simulink model "grasp_object"  (R2019a)
settings: Solver=FixedStepDiscrete  StartTime=0.0  StopTime=inf  FixedStep=0.001  RelTol=1e-3  EnableMultiTasking=on
PreLoadFcn:
  | demos_common_configs();
libraries: franka_simulink_library_misc x5, franka_simulink_library x3, simulink x1
settings Model: SimulationMode=external  ExtModeTrigDuration=10000  Creator=vasi_ko  LastModifiedBy=kvasios
settings DataIOCC: LimitDataPoints=on  SaveFormat=Array  ReturnWorkspaceOutputs=off
settings OptimizationCC: DefaultParameterBehavior=Inlined  EnhancedBackFolding=on  PassReuseOutputArgsAs=Individual arguments  ZeroExternalMemoryAtStartup=off  ZeroInternalMemoryAtStartup=off  OptimizeBlockOrder=speed  DifferentSizesBufferReuse=on  OptimizationCustomize=off
settings DebuggingCC: SolverPrmCheckMsg=warning  ParameterTunabilityLossMsg=error  SFUnexpectedBacktrackingDiag=warning  SFNoUnconditionalDefaultTransitionDiag=warning  SFExecutionAtInitializationDiag=none  ArithmeticOperatorsInVariantConditions=warning
settings HardwareCC: ProdBitPerLong=64  ProdHWDeviceType=Intel->x86-64 (Linux 64)
settings ModelReferenceCC: PropagateSignalLabelsOutOfModel=off
settings SFSimCC: SimUseLocalCustomCode=off  MATLABDynamicMemAlloc=off
settings RTWCC: SystemTargetFile=franka_emika_panda.tlc  GenCodeOnly=on  TemplateMakefile=ert_default_tmf  RTWVerbose=off  RTWUseLocalCustomCode=off  Toolchain=Franka Simulink | gmake (64-bit linux)  BuildConfiguration=Faster Runs  IncludeHyperlinkInReport=on  TargetLang=C++
settings CodeAppCC: ForceParamTrailComments=on  IgnoreCustomStorageClasses=off  OperatorAnnotations=on  SimulinkDataObjDesc=on  SFDataObjDesc=on  InsertBlockDesc=on
settings STFCustomTargetCC: TargetLangStandard=C99 (ISO)  MultiwordLength=256  GenerateSampleERTMain=on  ModelReferenceCompliant=off  CombineOutputUpdateFcns=on  ERTCustomFileBanners=on  SupportNonInlinedSFcns=off  RemoveResetFunc=on  MATLABClassNameForMDSCustomization=Simulink.SoftwareTarget.ERTCustomization  CPPClassGenCompliant=on  GRTInterface=off  UseToolchainInfoCompliant=on  SystemTargetFile=franka_emika_panda.tlc
settings ERTTargetCC: TargetLangStandard=C99 (ISO)  GenerateSampleERTMain=on  ModelReferenceCompliant=off  ParMdlRefBuildCompliant=off  CompOptLevelCompliant=off  ConcurrentExecutionCompliant=off  SupportContinuousTime=on  ModelStepFunctionPrototypeControlCompliant=off  InlinedParameterPlacement=NonHierarchical  ERTCustomFileTemplate=franka_emika_panda_file_process.tlc
settings ConfigComp: CovMetricSettings=dw  CovSaveCumulativeToWorkspaceVar=on  CovSaveSingleToWorkspaceVar=on  CovExternalEMLEnable=off  CovSFcnEnable=off

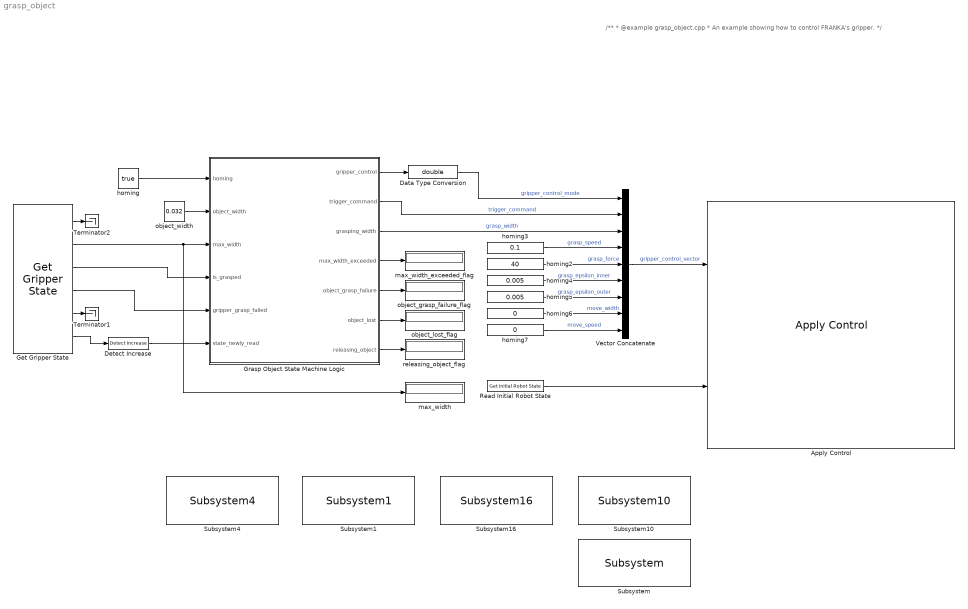
== system grasp_object ==
  note: /**
      |  * @example grasp_object.cpp
      |  * An example showing how to control FRANKA's gripper.
      |  */
  Apply Control : franka_simulink_library/Apply Control  robot_ip=robot_ip  gripper_attached=on  control_mode=Joint Positions - Internal Controller Mode  controller_choice=Joint Impedance Controller  elbow_control=on  collision_thresholds=100*ones(1,52)  joint_impedance=joint_impedance  cartesian_impedance=cartesian_impedance  load_inertia=load_inertia  EE_T_K=EE_T_K  init_joint_configuration_req=off  init_joint_configuration=q_init
      settings: SourceProductName=Franka Emika
  Data Type Conversion : DataTypeConversion  OutDataTypeStr=double
  Detect Increase : simulink/Logic and Bit Operations/Detect Increase  vinit=0.0  OutDataTypeStr=boolean
  Get Gripper State : franka_simulink_library/Get Gripper State  robot_ip=robot_ip
      settings: SourceProductName=Franka Emika
  Grasp Object State Machine Logic : Stateflow chart  TreatAsAtomicUnit=on
  Read Initial Robot State : franka_simulink_library/Get Initial Robot State  robot_ip=robot_ip  signals_requested='q_d'
      settings: SourceProductName=Franka Emika
  Subsystem : franka_simulink_library_misc/Subsystem  SystemSampleTime=-1  Latency=0  AutoFrameSizeCalculation=off
  Subsystem1 : franka_simulink_library_misc/Subsystem1  SystemSampleTime=-1  Latency=0  AutoFrameSizeCalculation=off
  Subsystem10 : franka_simulink_library_misc/Subsystem10  SystemSampleTime=-1  Latency=0  AutoFrameSizeCalculation=off
  Subsystem16 : franka_simulink_library_misc/Subsystem16  SystemSampleTime=-1  Latency=0  AutoFrameSizeCalculation=off
  Subsystem4 : franka_simulink_library_misc/Subsystem4  SystemSampleTime=-1  Latency=0  AutoFrameSizeCalculation=off
  Terminator1 : Terminator
  Terminator2 : Terminator
  Vector Concatenate : Concatenate  NumInputs=9
  homing : Constant  Value=true
  homing2 : Constant  Value=40
  homing3 : Constant  Value=0.1
  homing4 : Constant  Value=0.005
  homing5 : Constant  Value=0.005
  homing6 : Constant  Value=0
  homing7 : Constant  Value=0
  max_width : Display
  max_width_exceeded_flag : Display
  object_grasp_failure_flag : Display
  object_lost_flag : Display
  object_width : Constant  Value=0.032
  releasing_object_flag : Display
  wires:
  homing/1 -> Grasp Object State Machine Logic/1(homing)
  Get Gripper State/2 -> max_width/1, Grasp Object State Machine Logic/3(max_width)
  Get Gripper State/3 -> Grasp Object State Machine Logic/4(is_grasped)
  Read Initial Robot State/1 -> Apply Control/2
  Detect Increase/1 -> Grasp Object State Machine Logic/6(state_newly_read)
  Get Gripper State/6 -> Detect Increase/1
  Grasp Object State Machine Logic/1(gripper_control) -> Data Type Conversion/1
  Grasp Object State Machine Logic/4(max_width_exceeded) -> max_width_exceeded_flag/1
  Grasp Object State Machine Logic/5(object_grasp_failure) -> object_grasp_failure_flag/1
  Grasp Object State Machine Logic/6(object_lost) -> object_lost_flag/1
  Grasp Object State Machine Logic/7(releasing_object) -> releasing_object_flag/1
  Get Gripper State/4 -> Grasp Object State Machine Logic/5(gripper_grasp_failed)
  Get Gripper State/1 -> Terminator2/1
  Get Gripper State/5 -> Terminator1/1
  Vector Concatenate/1 -> Apply Control/1  "gripper_control_vector"
  Data Type Conversion/1 -> Vector Concatenate/1  "gripper_control_mode"
  Grasp Object State Machine Logic/3(grasping_width) -> Vector Concatenate/3  "grasp_width"
  homing3/1 -> Vector Concatenate/4  "grasp_speed"
  homing2/1 -> Vector Concatenate/5  "grasp_force"
  homing4/1 -> Vector Concatenate/6  "grasp_epsilon_inner"
  homing5/1 -> Vector Concatenate/7  "grasp_epsilon_outer"
  homing6/1 -> Vector Concatenate/8  "move_width"
  homing7/1 -> Vector Concatenate/9  "move_speed"
  object_width/1 -> Grasp Object State Machine Logic/2(object_width)
  Grasp Object State Machine Logic/2(trigger_command) -> Vector Concatenate/2  "trigger_command"

== stateflow chart grasp_object/Grasp Object State Machine Logic ==
  state starting_point
  state gripper_control_activated
  state homing
    en:gripper_control = gripper_control_modes.homing;
    trigger_command = trigger_command + 1;
  state read_state
    en:gripper_control = gripper_control_modes.read_state;
    trigger_command = trigger_command + 1;
  state max_grasp_width_check
  state max_grasp_width_within_range
    en:max_width_exceeded = 0;
  state max_grasp_width_exceeded
    en:max_width_exceeded = 1;
  state grasp_object
    en:grasping_width = object_width;
    gripper_control = gripper_control_modes.grasp;
    trigger_command = trigger_command + 1;
  state wait_grasp_command_update
  state grasp_succeeded
    en:object_grasp_failure = 0;
  state grasp_failed
    en:object_grasp_failure = 1;
  state read_state_2
    en:gripper_control = gripper_control_modes.read_state;
    trigger_command = trigger_command + 1;
  state check_if_object_is_lost
  state object_lost
    en:object_lost = 1;
  state object_not_lost
    en:object_lost = 0;
  state releasing_object
    en:gripper_control = gripper_control_modes.stop;
    trigger_command = trigger_command + 1;
  state fin
  (default) -> starting_point : {gripper_control = gripper_control_modes.idle;
      | trigger_command = 0;
      | max_width_exceeded = 0;
      | object_grasp_failure = 0;
      | object_lost=0;
      | releasing_object=0}
  starting_point -> gripper_control_activated : [state_newly_read]
  gripper_control_activated -> homing [order 1] : [homing]
  gripper_control_activated -> read_state [order 2] : [~homing]
  homing -> read_state : [state_newly_read]
  read_state -> max_grasp_width_check : [state_newly_read]
  max_grasp_width_check -> max_grasp_width_within_range [order 2] : [object_width<=max_width]
  max_grasp_width_check -> max_grasp_width_exceeded [order 1] : [object_width>max_width]
  max_grasp_width_within_range -> grasp_object : after(5,sec)
  grasp_object -> wait_grasp_command_update : [state_newly_read]
  wait_grasp_command_update -> grasp_failed [order 2] : [gripper_grasp_failed]
  wait_grasp_command_update -> grasp_succeeded [order 1] : [~gripper_grasp_failed]
  grasp_succeeded -> read_state_2 : after(3,sec)
  read_state_2 -> check_if_object_is_lost : [state_newly_read]
  check_if_object_is_lost -> object_lost [order 1] : [~is_grasped]
  check_if_object_is_lost -> object_not_lost [order 2] : [is_grasped]
  object_not_lost -> releasing_object : {releasing_object = 1;}
  releasing_object -> fin : [state_newly_read]
  data: gripper_control output; trigger_command output; grasping_width output; homing input; object_width input; max_width input; is_grasped input; gripper_grasp_failed input; state_newly_read input; max_width_exceeded output; object_grasp_failure output; object_lost output; releasing_object output
